simulink model "HANcoder_E407_DYS_MP"  (R2018b)
settings: Solver=FixedStepDiscrete  StartTime=0.0  StopTime=1  FixedStep=0.01  RelTol=1e-3
PreLoadFcn:
  | librarySetup
  | eval([bdroot,'_startup']) %Calling [modelName]_startup.m
values from neighbouring files (symbols this model uses):
  basic_cycle_duration_bc0 = TM_Reset_Board   + COMP_duration    (= 212)    [HANcoder_E407_DYS_MP_startup.m]
  basic_cycle_duration_bc1 = basic_cycle_duration_bc0    (= 212)    [HANcoder_E407_DYS_MP_startup.m]
  comm_delay_estimation1 = round(comm_delay_measured1*hardware_granularity/frequency_IRQ)    [HANcoder_E407_DYS_MP_startup.m]
  comm_delay_estimation2 = round(comm_delay_measured2*hardware_granularity/frequency_IRQ)    [HANcoder_E407_DYS_MP_startup.m]
  COMM_Phase1 = Simulink.Parameter    [HANcoder_E407_DYS_MP_startup.m]
  COMM_Phase2 = Simulink.Parameter    [HANcoder_E407_DYS_MP_startup.m]
  frequency_IRQ = 500    [HANcoder_E407_DYS_MP_startup.m]
  HantuneAngleSp = Simulink.Parameter    [HANcoder_E407_DYS_MP_startup.m]
  idle_time_init = basic_cycle_duration_bc0 + basic_cycle_duration_bc1    (= 424)    [HANcoder_E407_DYS_MP_startup.m]
  matrix_rows = 2    [HANcoder_E407_DYS_MP_startup.m]
  positionD = Simulink.Parameter    [HANcoder_E407_DYS_MP_startup.m]
  positionI = Simulink.Parameter    [HANcoder_E407_DYS_MP_startup.m]
  positionP = Simulink.Parameter    [HANcoder_E407_DYS_MP_startup.m]
undefined symbols (not defined in the file or in its folder): A1, CON2, CON4, D13, Dposition, Iposition, Pposition
libraries: HANcoder_STM32_Target x33, dspswit3 x16, simulink x2, simulink_extras x2, dspstat3 x1
(part 2 of 10)

== system HANcoder_E407_DYS_MP/HANcoder STM32 Target - E407-STM32 algorithm/4.TTA Can System/4.3 TTA System/4.3.1 Initialization/Receive can message ==
  Can_ID : Inport
  Action Port : ActionPort  ActionType=then
  CAN receive : Subsystem  Tag=HANcoder_TARGET_STM32_E407  AncestorBlock=HANcoder_STM32_Target/STM32-E407/CAN/CAN/CAN receive  mask(CAN receive){canBus=CAN 1, outputNumber=1, dataType=uint8, byteOrder=off, tsamp=-1}
      mask prompts: canBus "CAN channel"; outputNumber "Output ports"; dataType "Output datatype"; byteOrder "Byte order: Checked = MSB first, unchecked = LSB first."; tsamp "Sample time"
      mask help:
      | Function
      | ==========
      | Receive the newest message from the specified CAN channel.
      |
      | Parameters
      | ==========
      | CAN channel:             The CAN channel to send the message on.
      | Output ports:             The amount of output ports
      | Output datatype:       The datatype of the output ports
      | Byte order:                 Select MSB or LSB first
      | Sample time:              -1 or divisible by base sample time [seconds]
      |
      | Input
      | ==========
      | Port 1:                       CAN ID(uint32) in hexadecimal ie: hex2dec('0a')
      |
      | Output
      | ==========
      | Port 1:                       Checks for new message(int8)
      | Port 2..9                     Message data
      mask init:
      | sfcn_can_receive_mcb(canBus, outputNumber, dataType, byteOrder)
      settings: MoveFcn=drawLogos
      mask Help: web('sfcn_can_receive.html');
      mask TypeOptions canBus: CAN 1 | CAN 2
      mask TypeOptions dataType: int8 | uint8 | int16 | uint16 | int32 | uint32 | boolean
      mask Display:
      | fprintf('Receive on\nCAN %x', canBus);
      | port_label('output', 1, 'new');
      | port_label('input', 1, 'ID');patch([75 81 81],[8 14 2],[1 0 0]);patch([83 83 89],[14 2 8],[0 0 0.35]);
  CAN receive2 : Subsystem  Tag=HANcoder_TARGET_STM32_E407  AncestorBlock=HANcoder_STM32_Target/STM32-E407/CAN/CAN/CAN receive  mask(CAN receive){canBus=CAN 2, outputNumber=1, dataType=uint8, byteOrder=off, tsamp=-1}
      mask prompts: canBus "CAN channel"; outputNumber "Output ports"; dataType "Output datatype"; byteOrder "Byte order: Checked = MSB first, unchecked = LSB first."; tsamp "Sample time"
      mask help:
      | Function
      | ==========
      | Receive the newest message from the specified CAN channel.
      |
      | Parameters
      | ==========
      | CAN channel:             The CAN channel to send the message on.
      | Output ports:             The amount of output ports
      | Output datatype:       The datatype of the output ports
      | Byte order:                 Select MSB or LSB first
      | Sample time:              -1 or divisible by base sample time [seconds]
      |
      | Input
      | ==========
      | Port 1:                       CAN ID(uint32) in hexadecimal ie: hex2dec('0a')
      |
      | Output
      | ==========
      | Port 1:                       Checks for new message(int8)
      | Port 2..9                     Message data
      mask init:
      | sfcn_can_receive_mcb(canBus, outputNumber, dataType, byteOrder)
      settings: MoveFcn=drawLogos
      mask Help: web('sfcn_can_receive.html');
      mask TypeOptions canBus: CAN 1 | CAN 2
      mask TypeOptions dataType: int8 | uint8 | int16 | uint16 | int32 | uint32 | boolean
      mask Display:
      | fprintf('Receive on\nCAN %x', canBus);
      | port_label('output', 1, 'new');
      | port_label('input', 1, 'ID');patch([75 81 81],[8 14 2],[1 0 0]);patch([83 83 89],[14 2 8],[0 0 0.35]);
  Can1Mes1 : Outport
  Can1Receive : Outport  Port=2
  Can2Mes2 : Outport  Port=3
  Can2Receive : Outport  Port=4
  wires:
  CAN receive/2(Out2) -> Can1Mes1/1  "Test_CanMes0"
  CAN receive/1(Out1) -> Can1Receive/1  "Test_CanRec529"
  Can_ID/1 -> CAN receive2/1(In1), CAN receive/1(In1)
  CAN receive2/1(Out1) -> Can2Receive/1  "Test_Can2Rec529"
  CAN receive2/2(Out2) -> Can2Mes2/1  "Test_CanMes2"

== system HANcoder_E407_DYS_MP/HANcoder STM32 Target - E407-STM32 algorithm/4.TTA Can System/4.3 TTA System/4.3.1 Initialization/RoleID and Global Time init ==
  note: Reset variables
  note: Finish Initialization
  note: Role_ID Initialization
  Timeout Initialization : Inport
  Reference message received : Inport  Port=2
  Can1_Mes : Inport  Port=3
  Can1_New : Inport  Port=4
  Can2_Mes1 : Inport  Port=5
  Can2_New : Inport  Port=6
  Enable : EnablePort
  Constant : Constant  Priority=4
  Constant1 : Constant  Priority=3  Value=2
  Data Store Read : DataStoreRead  Priority=5  DataStoreName=Role_ID
  Data Store Write : DataStoreWrite  Priority=8  DataStoreName=Role_ID
  Data Store Write2 : DataStoreWrite  Priority=18  DataStoreName=Delay_Counter
  Data Store Write4 : DataStoreWrite  Priority=16  DataStoreName=Initialization_Timeout
  Global Time Initialization Master : Subsystem  Priority=2
  Global Time Initialization Slave : Subsystem  Priority=1
  RESET : Constant  Priority=15  Value=0  OutDataTypeStr=boolean
  RESET1 : Constant  Priority=17  Value=0  OutDataTypeStr=double
  SET : Constant  Priority=19
  Switch1 : Switch  Priority=6  Criteria=u2 > Threshold
  Switch2 : Switch  Priority=7  Criteria=u2 > Threshold
  Finish Initialization : Outport  OutputWhenDisabled=reset  InitialOutput=0
  wires:
  Switch1/1 -> Switch2/3
  Reference message received/1 -> Switch2/2, Global Time Initialization Slave/Enable  "Check"
  Data Store Read/1 -> Switch1/3
  SET/1 -> Finish Initialization/1
  Constant/1 -> Switch1/1
  Constant1/1 -> Switch2/1
  Switch2/1 -> Data Store Write/1
  RESET/1 -> Data Store Write4/1
  Timeout Initialization/1 -> Switch1/2, Global Time Initialization Master/Enable
  RESET1/1 -> Data Store Write2/1
  Can1_Mes/1 -> Global Time Initialization Slave/1(Can1_Mes)
  Can1_New/1 -> Global Time Initialization Slave/2(Can1_New)
  Can2_Mes1/1 -> Global Time Initialization Slave/3(Can2_Mes1)
  Can2_New/1 -> Global Time Initialization Slave/4(Can2_New)

== system HANcoder_E407_DYS_MP/HANcoder STM32 Target - E407-STM32 algorithm/4.TTA Can System/4.3 TTA System/4.3.3 Matrix Cycle Manager/4.3.3.1 Controller Matrix Cycle Truck Boards 1 2 and 3 ==
  note: Nodes Voting
      | Own_Vote:
      |    Individual vote of current node
      |
      |
      | Votes_count:
      |    Count of all received votes
  Enable : EnablePort  PropagateVarSize=During execution
  4.3.3.1.1 controller basic cycle 0.1 : Subsystem
  4.3.3.1.2 controller basic cycle 0.2 : Subsystem
  Data Store Memory : DataStoreMemory  DataStoreName=msg_count_DEBUG  ReadBeforeWriteMsg=warning  WriteAfterWriteMsg=warning  WriteAfterReadMsg=warning  ShowAdditionalParam=off
  Data Store Memory1 : DataStoreMemory  DataStoreName=Board1_error_counter  ReadBeforeWriteMsg=warning  WriteAfterWriteMsg=warning  WriteAfterReadMsg=warning  ShowAdditionalParam=off  OutMin=0  OutMax=4294967294  OutDataTypeStr=double
  Data Store Memory10 : DataStoreMemory  DataStoreName=Sensor_missed_counter  ReadBeforeWriteMsg=warning  WriteAfterWriteMsg=warning  WriteAfterReadMsg=warning  ShowAdditionalParam=off  OutMin=0  OutMax=4294967294  OutDataTypeStr=double
  Data Store Memory11 : DataStoreMemory  DataStoreName=Out1_missed_counter  ReadBeforeWriteMsg=warning  WriteAfterWriteMsg=warning  WriteAfterReadMsg=warning  ShowAdditionalParam=off  OutMin=0  OutMax=4294967294  OutDataTypeStr=double
  Data Store Memory12 : DataStoreMemory  Priority=30  DataStoreName=Own_Vote  ReadBeforeWriteMsg=warning  WriteAfterWriteMsg=warning  WriteAfterReadMsg=warning  ShowAdditionalParam=off  OutDataTypeStr=uint8
  Data Store Memory13 : DataStoreMemory  DataStoreName=Sync_bc1_missed_counter  ReadBeforeWriteMsg=warning  WriteAfterWriteMsg=warning  WriteAfterReadMsg=warning  ShowAdditionalParam=off  OutMin=0  OutMax=4294967294  OutDataTypeStr=double
  Data Store Memory14 : DataStoreMemory  DataStoreName=Out2_missed_counter  ReadBeforeWriteMsg=warning  WriteAfterWriteMsg=warning  WriteAfterReadMsg=warning  ShowAdditionalParam=off  OutMin=0  OutMax=4294967294  OutDataTypeStr=double
  Data Store Memory15 : DataStoreMemory  DataStoreName=NoMes1Cnt  ReadBeforeWriteMsg=warning  WriteAfterWriteMsg=warning  WriteAfterReadMsg=warning  ShowAdditionalParam=off  OutMin=0  OutMax=4294967294  OutDataTypeStr=double
  Data Store Memory16 : DataStoreMemory  DataStoreName=NoMes2Cnt  ReadBeforeWriteMsg=warning  WriteAfterWriteMsg=warning  WriteAfterReadMsg=warning  ShowAdditionalParam=off  OutMin=0  OutMax=4294967294  OutDataTypeStr=double
  Data Store Memory17 : DataStoreMemory  DataStoreName=NoMes3Cnt  ReadBeforeWriteMsg=warning  WriteAfterWriteMsg=warning  WriteAfterReadMsg=warning  ShowAdditionalParam=off  OutMin=0  OutMax=4294967294  OutDataTypeStr=double
  Data Store Memory18 : DataStoreMemory  DataStoreName=CycleCnt  ReadBeforeWriteMsg=warning  WriteAfterWriteMsg=warning  WriteAfterReadMsg=warning  ShowAdditionalParam=off  OutMin=0  OutMax=4294967294  OutDataTypeStr=double
  Data Store Memory19 : DataStoreMemory  DataStoreName=VoteTime  ReadBeforeWriteMsg=warning  WriteAfterWriteMsg=warning  WriteAfterReadMsg=warning  ShowAdditionalParam=off  OutMin=0  OutMax=250  OutDataTypeStr=uint8
  Data Store Memory2 : DataStoreMemory  DataStoreName=Board2_error_counter  ReadBeforeWriteMsg=warning  WriteAfterWriteMsg=warning  WriteAfterReadMsg=warning  ShowAdditionalParam=off  OutMin=0  OutMax=4294967294  OutDataTypeStr=double
  Data Store Memory20 : DataStoreMemory  DataStoreName=NoMes1  ReadBeforeWriteMsg=warning  WriteAfterWriteMsg=warning  WriteAfterReadMsg=warning  ShowAdditionalParam=off  OutMin=0  OutMax=4294967294  OutDataTypeStr=double
  Data Store Memory21 : DataStoreMemory  DataStoreName=NoMes2  ReadBeforeWriteMsg=warning  WriteAfterWriteMsg=warning  WriteAfterReadMsg=warning  ShowAdditionalParam=off  OutMin=0  OutMax=4294967294  OutDataTypeStr=double
  Data Store Memory22 : DataStoreMemory  DataStoreName=NoMes3  ReadBeforeWriteMsg=warning  WriteAfterWriteMsg=warning  WriteAfterReadMsg=warning  ShowAdditionalParam=off  OutMin=0  OutMax=4294967294  OutDataTypeStr=double
  Data Store Memory3 : DataStoreMemory  DataStoreName=Board3_error_counter  ReadBeforeWriteMsg=warning  WriteAfterWriteMsg=warning  WriteAfterReadMsg=warning  ShowAdditionalParam=off  OutMin=0  OutMax=4294967294  OutDataTypeStr=double
  Data Store Memory4 : DataStoreMemory  Priority=30  DataStoreName=BC0_Vote2_processed  ReadBeforeWriteMsg=warning  WriteAfterWriteMsg=warning  WriteAfterReadMsg=warning  ShowAdditionalParam=off  OutDataTypeStr=boolean
  Data Store Memory5 : DataStoreMemory  Priority=30  DataStoreName=BC0_Vote3_processed  ReadBeforeWriteMsg=warning  WriteAfterWriteMsg=warning  WriteAfterReadMsg=warning  ShowAdditionalParam=off  OutDataTypeStr=boolean
  Data Store Memory6 : DataStoreMemory  Priority=30  DataStoreName=BC0_Vote1_processed  ReadBeforeWriteMsg=warning  WriteAfterWriteMsg=warning  WriteAfterReadMsg=warning  ShowAdditionalParam=off  OutDataTypeStr=boolean
  Data Store Memory7 : DataStoreMemory  DataStoreName=Sync_bc0_missed_counter  ReadBeforeWriteMsg=warning  WriteAfterWriteMsg=warning  WriteAfterReadMsg=warning  ShowAdditionalParam=off  OutMin=0  OutMax=4294967294  OutDataTypeStr=double
  Data Store Memory8 : DataStoreMemory  DataStoreName=Set_missed_counter  ReadBeforeWriteMsg=warning  WriteAfterWriteMsg=warning  WriteAfterReadMsg=warning  ShowAdditionalParam=off  OutMin=0  OutMax=4294967294  OutDataTypeStr=double
  Data Store Memory9 : DataStoreMemory  Priority=30  DataStoreName=Votes_count  ReadBeforeWriteMsg=warning  WriteAfterWriteMsg=warning  WriteAfterReadMsg=warning  ShowAdditionalParam=off  OutDataTypeStr=Bus: vote_array
  Matrix_Cycle_Observation_DEBUG : Subsystem
  msg_count_DEBUG observer : Subsystem

== system HANcoder_E407_DYS_MP/HANcoder STM32 Target - E407-STM32 algorithm/4.TTA Can System/4.3 TTA System/4.3.3 Matrix Cycle Manager/4.3.3.2 Controller Matrix Cycle_Board 4 and 5 ==
  Enable : EnablePort  PropagateVarSize=During execution
  controller basic cycle 0 : Subsystem
  controller basic cycle 0.2 : Subsystem

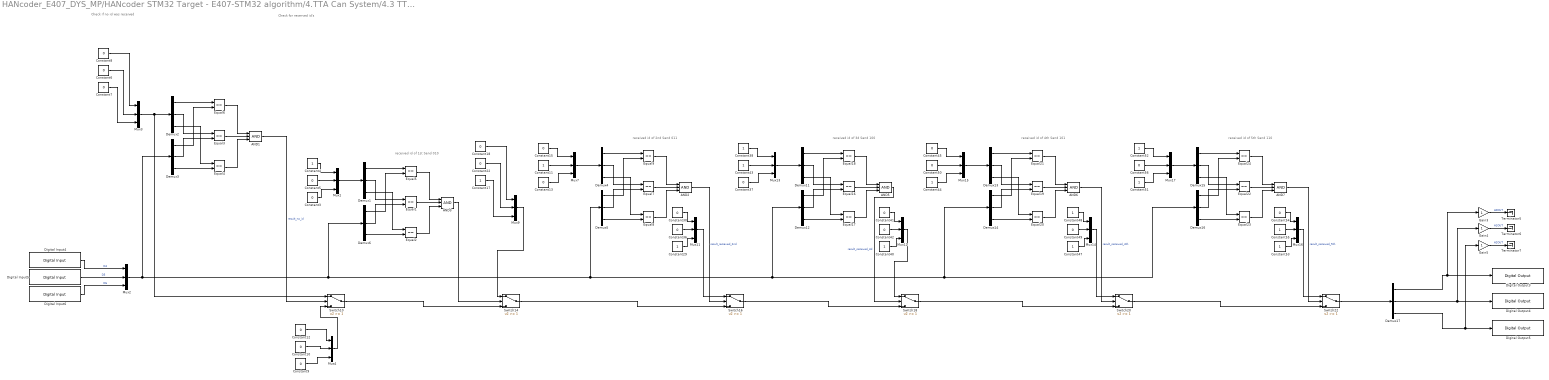
== system HANcoder_E407_DYS_MP/HANcoder STM32 Target - E407-STM32 algorithm/4.TTA Can System/4.3 TTA System/4.3.3 Matrix Cycle Manager/4.3.3.3 Send the next Board ID ==
  note: received id of 2nd
      | Send 011
  note: received id of 3d
      | Send 100
  note: received id of 4th
      | Send 101
  note: received id of 5th
      | Send 110
  note: Check if no id was received
  note: received id of 1st
      | Send 010
  note: Check for reserved id's
  AND{1..3,5..7} (6 alike) : Logic  Inputs=3  AllPortsSameDT=off  OutDataTypeStr=boolean
  Constant{3,5..10,12..13,15,18,22,30,36..37,41..42,45,49..50,54,56} (22 alike) : Constant  Value=0  OutDataTypeStr=boolean
  Constant{4,11,17,29,38,40,43..44,47..48,51..53,55} (14 alike) : Constant  OutDataTypeStr=boolean
  Demux{1..6,11..17} (13 alike) : Demux  Outputs=3
  Digital Input4 : HANcoder_STM32_Target/STM32-E407/Digital Inputs/Digital Input  Tag=HANcoder_TARGET_STM32_E407  pinID=CON3 - D2 - 5V Tolerant  config=Pulldown  tsamp=-1
      settings: SourceProductName=HANcoder STM32 Target
  Digital Input5 : HANcoder_STM32_Target/STM32-E407/Digital Inputs/Digital Input  Tag=HANcoder_TARGET_STM32_E407  pinID=CON3 - D3 - 5V Tolerant  config=Pulldown  tsamp=-1
      settings: SourceProductName=HANcoder STM32 Target
  Digital Input6 : HANcoder_STM32_Target/STM32-E407/Digital Inputs/Digital Input  Tag=HANcoder_TARGET_STM32_E407  pinID=CON3 - D4 - 5V Tolerant  config=Pulldown  tsamp=-1
      settings: SourceProductName=HANcoder STM32 Target
  Digital Output3 : HANcoder_STM32_Target/STM32-E407/Digital Outputs/Digital Output  Tag=HANcoder_TARGET_STM32_E407  pinID=CON PD - 8  config=Push pull  tsamp=-1
      settings: SourceProductName=HANcoder STM32 Target
  Digital Output4 : HANcoder_STM32_Target/STM32-E407/Digital Outputs/Digital Output  Tag=HANcoder_TARGET_STM32_E407  pinID=CON PD - 9  config=Push pull  tsamp=-1
      settings: SourceProductName=HANcoder STM32 Target
  Digital Output5 : HANcoder_STM32_Target/STM32-E407/Digital Outputs/Digital Output  Tag=HANcoder_TARGET_STM32_E407  pinID=CON PD - 10  config=Push pull  tsamp=-1
      settings: SourceProductName=HANcoder STM32 Target
  Equal{1..9,16..24} (18 alike) : RelationalOperator  Operator===  OutDataTypeStr=boolean  RndMeth=Simplest
  Gain3 : Gain
  Gain4 : Gain
  Gain5 : Gain
  Mux{1..4,7,9,11..17} (13 alike) : Mux  Inputs=3
  Switch{10,14,16,18,20,22} (6 alike) : Switch  Threshold=1
  Terminator5 : Terminator
  Terminator6 : Terminator
  Terminator7 : Terminator
  wires:
  Switch14/1 -> Switch16/3
  Constant29/1 -> Mux11/3
  Constant36/1 -> Mux11/2
  Constant17/1 -> Mux9/3
  Demux5/3 -> Equal8/2
  Mux9/1 -> Switch14/1
  Demux4/1 -> Equal9/1
  Demux5/2 -> Equal7/2
  Equal3/1 -> AND1/2
  Mux2/1 -> Demux3/1, Demux6/1, Demux5/1, Demux16/1, Demux14/1, Demux12/1
  Mux7/1 -> Demux4/1
  Demux4/2 -> Equal7/1
  Constant13/1 -> Mux7/3
  Demux2/2 -> Equal3/1
  Digital Input5/1 -> Mux2/2  "D5"
  Digital Input6/1 -> Mux2/3  "D6"
  Demux3/2 -> Equal3/2
  Constant41/1 -> Mux12/1
  AND2/1 -> Switch16/2  "result_recieved_2nd"
  Constant7/1 -> Mux3/3
  Constant51/1 -> Mux17/3
  Demux3/3 -> Equal4/2
  AND1/1 -> Switch10/2  "result_no_id"
  Demux15/2 -> Equal22/1
  Demux5/1 -> Equal9/2
  Switch22/1 -> Demux17/1
  Demux16/1 -> Equal24/2
  Equal9/1 -> AND2/1
  Mux15/1 -> Demux13/1
  Demux17/3 -> Gain5/1, Digital Output5/1
  Gain4/1 -> Terminator6/1  "A1OUT"
  Equal22/1 -> AND7/2
  Switch10/1 -> Switch14/3
  Constant12/1 -> Mux4/1
  Constant10/1 -> Mux4/2
  Constant9/1 -> Mux4/3
  Demux11/2 -> Equal16/1
  Demux14/1 -> Equal21/2
  Constant11/1 -> Mux7/2
  Switch18/1 -> Switch20/3
  Equal16/1 -> AND5/2
  Constant53/1 -> Mux16/3
  Equal6/1 -> AND1/1
  Demux12/1 -> Equal18/2
  Gain5/1 -> Terminator7/1  "A2OUT"
  Constant55/1 -> Mux16/2
  Mux16/1 -> Switch22/1
  Gain3/1 -> Terminator5/1  "A0OUT"
  Equal7/1 -> AND2/2
  Demux2/1 -> Equal6/1
  Demux15/3 -> Equal23/1
  Demux16/3 -> Equal23/2
  AND6/1 -> Switch20/2  "result_recieved_4th"
  Demux15/1 -> Equal24/1
  Switch20/1 -> Switch22/3
  Demux2/3 -> Equal4/1
  Demux16/2 -> Equal22/2
  Constant56/1 -> Mux17/2
  Mux14/1 -> Switch20/1
  Mux17/1 -> Demux15/1
  Demux17/1 -> Gain3/1, Digital Output3/1
  Constant37/1 -> Mux13/3
  Constant42/1 -> Mux12/2
  Constant6/1 -> Mux3/2
  Demux13/2 -> Equal19/1
  Demux4/3 -> Equal8/1
  Constant18/1 -> Mux9/1
  Constant8/1 -> Mux3/1
  Constant44/1 -> Mux15/3
  Constant49/1 -> Mux14/2
  Demux11/1 -> Equal18/1
  Constant47/1 -> Mux14/3
  Equal23/1 -> AND7/3
  Switch16/1 -> Switch18/3
  Constant40/1 -> Mux12/3
  Constant52/1 -> Mux17/1
  Constant38/1 -> Mux13/1
  Constant15/1 -> Mux7/1
  Constant22/1 -> Mux9/2
  Constant45/1 -> Mux15/1
  Equal4/1 -> AND1/3
  Mux3/1 -> Demux2/1, Switch10/1
  Mux11/1 -> Switch16/1
  Demux14/3 -> Equal20/2
  Demux12/3 -> Equal17/2
  Mux12/1 -> Switch18/1
  Equal24/1 -> AND7/1
  Demux11/3 -> Equal17/1
  Demux12/2 -> Equal16/2
  Equal19/1 -> AND6/2
  Demux13/3 -> Equal20/1
  AND5/1 -> Switch18/2  "result_recieved_3d"
  Demux17/2 -> Gain4/1, Digital Output4/1
  Constant43/1 -> Mux13/2
  Digital Input4/1 -> Mux2/1  "D4"
  Constant4/1 -> Mux1/1
  Equal17/1 -> AND5/3
  Demux14/2 -> Equal19/2
  Constant50/1 -> Mux15/2
  Demux3/1 -> Equal6/2
  Demux1/3 -> Equal2/1
  Constant54/1 -> Mux16/1
  Equal1/1 -> AND3/2
  Equal20/1 -> AND6/3
  Constant5/1 -> Mux1/2
  Equal2/1 -> AND3/3
  Constant3/1 -> Mux1/3
  Constant48/1 -> Mux14/1
  Demux1/2 -> Equal1/1
  Mux1/1 -> Demux1/1
  Constant30/1 -> Mux11/1
  Mux13/1 -> Demux11/1
  Equal18/1 -> AND5/1
  Demux1/1 -> Equal5/1
  AND7/1 -> Switch22/2  "result_recieved_5th"
  Demux6/3 -> Equal2/2
  Demux13/1 -> Equal21/1
  Equal21/1 -> AND6/1
  Demux6/1 -> Equal5/2
  Equal8/1 -> AND2/3
  Mux4/1 -> Switch10/3
  Demux6/2 -> Equal1/2
  Equal5/1 -> AND3/1
  AND3/1 -> Switch14/2

== system HANcoder_E407_DYS_MP/HANcoder STM32 Target - E407-STM32 algorithm/4.TTA Can System/4.3 TTA System/4.3.3 Matrix Cycle Manager/Matrix_Cycle_Observation_DEBUG ==
  Data Store Read1 : DataStoreRead  DataStoreName=TrailerOneAttachedFlag
  Data Store Read17 : DataStoreRead  DataStoreName=Votes_Angle  DataStoreElements=Votes_Angle.First_Board#Votes_Angle.Second_Board#Votes_Angle.Third_Board
  Data Store Read18 : DataStoreRead  DataStoreName=InputAngle1
  Data Store Read2 : DataStoreRead  DataStoreName=TwoTrailersAttachedFlag
  Data Store Read3 : DataStoreRead  DataStoreName=InputAngle2
  Data Store Read4 : DataStoreRead  DataStoreName=Votes_Encoder  DataStoreElements=Votes_Encoder.First_Board#Votes_Encoder.Second_Board#Votes_Encoder.Third_Board
  Terminator{1..6,19..22} (10 alike) : Terminator
  wires:
  Data Store Read18/1 -> Terminator22/1  "InputAngleBoard4"
  Data Store Read17/3 -> Terminator21/1  "VoteAngle3"
  Data Store Read17/2 -> Terminator20/1  "VoteAngle2"
  Data Store Read17/1 -> Terminator19/1  "VoteAngle1"
  Data Store Read1/1 -> Terminator1/1  "TrailerOneAttach"
  Data Store Read2/1 -> Terminator2/1  "TrailerTwoAttach"
  Data Store Read3/1 -> Terminator3/1  "InputAngleBoard5"
  Data Store Read4/1 -> Terminator4/1  "VoteEncoder1"
  Data Store Read4/3 -> Terminator6/1  "VoteEncoder3"
  Data Store Read4/2 -> Terminator5/1  "VoteEncoder2"

== system HANcoder_E407_DYS_MP/HANcoder STM32 Target - E407-STM32 algorithm/4.TTA Can System/4.3 TTA System/4.3.1 Initialization/Receive can message/CAN receive ==
  In1 : Inport
  Enabled Subsystem : Subsystem  TreatAsAtomicUnit=on
  S-Function : M-S-Function  FunctionName=sfcn_can_receive  Parameters=tsamp, canBus, outputNumber, dataType, byteOrder
  Term{3..9} (7 alike) : Terminator
  Out1 : Outport
  Out2 : Outport  Port=2
  wires:
  S-Function/9 -> Enabled Subsystem/8(In8)
  S-Function/4 -> Enabled Subsystem/3(In3)
  S-Function/5 -> Enabled Subsystem/4(In4)
  S-Function/8 -> Enabled Subsystem/7(In7)
  S-Function/7 -> Enabled Subsystem/6(In6)
  S-Function/6 -> Enabled Subsystem/5(In5)
  Enabled Subsystem/8(Out8) -> Term9/1
  Enabled Subsystem/7(Out7) -> Term8/1
  Enabled Subsystem/6(Out6) -> Term7/1
  Enabled Subsystem/5(Out5) -> Term6/1
  Enabled Subsystem/4(Out4) -> Term5/1
  Enabled Subsystem/3(Out3) -> Term4/1
  Enabled Subsystem/2(Out2) -> Term3/1
  Enabled Subsystem/1(Out1) -> Out2/1
  S-Function/3 -> Enabled Subsystem/2(In2)
  S-Function/2 -> Enabled Subsystem/1(In1)
  S-Function/1 -> Out1/1, Enabled Subsystem/Enable
  In1/1 -> S-Function/1

== system HANcoder_E407_DYS_MP/HANcoder STM32 Target - E407-STM32 algorithm/4.TTA Can System/4.3 TTA System/4.3.1 Initialization/Receive can message/CAN receive2 ==
  In1 : Inport
  Enabled Subsystem : Subsystem  TreatAsAtomicUnit=on
  S-Function : M-S-Function  FunctionName=sfcn_can_receive  Parameters=tsamp, canBus, outputNumber, dataType, byteOrder
  Term{3..9} (7 alike) : Terminator
  Out1 : Outport
  Out2 : Outport  Port=2
  wires:
  S-Function/9 -> Enabled Subsystem/8(In8)
  S-Function/4 -> Enabled Subsystem/3(In3)
  S-Function/5 -> Enabled Subsystem/4(In4)
  S-Function/8 -> Enabled Subsystem/7(In7)
  S-Function/7 -> Enabled Subsystem/6(In6)
  S-Function/6 -> Enabled Subsystem/5(In5)
  Enabled Subsystem/8(Out8) -> Term9/1
  Enabled Subsystem/7(Out7) -> Term8/1
  Enabled Subsystem/6(Out6) -> Term7/1
  Enabled Subsystem/5(Out5) -> Term6/1
  Enabled Subsystem/4(Out4) -> Term5/1
  Enabled Subsystem/3(Out3) -> Term4/1
  Enabled Subsystem/2(Out2) -> Term3/1
  Enabled Subsystem/1(Out1) -> Out2/1
  S-Function/3 -> Enabled Subsystem/2(In2)
  S-Function/2 -> Enabled Subsystem/1(In1)
  S-Function/1 -> Out1/1, Enabled Subsystem/Enable
  In1/1 -> S-Function/1

== system HANcoder_E407_DYS_MP/HANcoder STM32 Target - E407-STM32 algorithm/4.TTA Can System/4.3 TTA System/4.3.1 Initialization/RoleID and Global Time init/Global Time Initialization Master ==
  note: Global Time Initialization
  Enable : EnablePort
  Board nr1 : Constant
  Cast : DataTypeConversion  OutDataTypeStr=uint16
  Cast1 : DataTypeConversion  OutDataTypeStr=uint8
  Data Store Write : DataStoreWrite  DataStoreName=Local_Ticks
  Data Store Write1 : DataStoreWrite  DataStoreName=basic_cycle_count
  Data Store Write3 : DataStoreWrite  DataStoreName=Master_ID
  Start : Constant  Value=0
  wires:
  Board nr1/1 -> Data Store Write3/1
  Start/1 -> Cast1/1, Cast/1
  Cast/1 -> Data Store Write/1
  Cast1/1 -> Data Store Write1/1

== system HANcoder_E407_DYS_MP/HANcoder STM32 Target - E407-STM32 algorithm/4.TTA Can System/4.3 TTA System/4.3.1 Initialization/RoleID and Global Time init/Global Time Initialization Slave ==
  note: Sync has already been received, so we skip
      | the first comp tasks related to Update LT.
  note: Global Time Initialization
  Can1_Mes : Inport
  Can1_New : Inport  Port=2
  Can2_Mes1 : Inport  Port=3
  Can2_New : Inport  Port=4
  Enable : EnablePort
  Cast1 : DataTypeConversion  OutDataTypeStr=double
  Constant : Constant  Value=25  OutDataTypeStr=uint16
  Constant1 : Constant  Commented=on  Value=COMM_Phase1
  Constant2 : Constant  Commented=on  Value=COMM_Phase2
  Constant3 : Constant  Value=25  OutDataTypeStr=uint16
  Constant4 : Constant  Value=0  OutDataTypeStr=uint8
  Data Store Read : DataStoreRead  Priority=5  DataStoreName=Board_ID
  Data Store Write1 : DataStoreWrite  DataStoreName=Local_Ticks
  Data Store Write2 : DataStoreWrite  DataStoreName=basic_cycle_count
  Data Store Write3 : DataStoreWrite  DataStoreName=Master_ID
  Data Store Write4 : DataStoreWrite  Priority=10  DataStoreName=BC0_Sync_processed
  Data Type Conversion : DataTypeConversion  Commented=on  OutDataTypeStr=uint16
  Data Type Conversion1 : DataTypeConversion  Commented=on  OutDataTypeStr=uint16
  "SET1 " : Constant  Priority=9  OutDataTypeStr=boolean
  Sum : Sum  Priority=11  Inputs=+++  AccumDataTypeStr=uint16
  Sum1 : Sum  Priority=13  Inputs=+++  AccumDataTypeStr=uint16
  Switch1 : Switch  Priority=22  Criteria=u2 > Threshold
  delay_estimation_1 : Constant  Value=comm_delay_estimation1  OutDataTypeStr=uint16
  delay_estimation_2 : Constant  Value=comm_delay_estimation2  OutDataTypeStr=uint16
  wires:
  "SET1 "/1 -> Data Store Write4/1
  Switch1/1 -> Data Store Write1/1  "Rx_init_LT_Init"
  Cast1/1 -> Data Store Write3/1
  Constant/1 -> Sum/2
  delay_estimation_2/1 -> Sum1/3
  delay_estimation_1/1 -> Sum/3
  Can1_New/1 -> Switch1/2
  Sum/1 -> Switch1/1  "EstimatedTimeCan1_Init"
  Constant3/1 -> Sum1/2
  Sum1/1 -> Switch1/3  "EstimatedTimeCan2_Init"
  Constant4/1 -> Data Store Write2/1
  Data Store Read/1 -> Cast1/1
  Constant1/1 -> Data Type Conversion/1
  Data Type Conversion/1 -> Sum/1
  Constant2/1 -> Data Type Conversion1/1
  Data Type Conversion1/1 -> Sum1/1

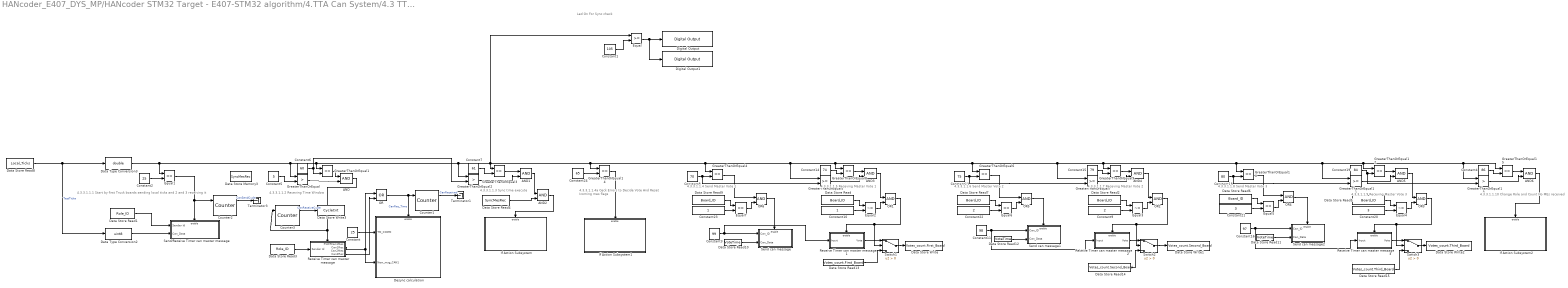
== system HANcoder_E407_DYS_MP/HANcoder STM32 Target - E407-STM32 algorithm/4.TTA Can System/4.3 TTA System/4.3.3 Matrix Cycle Manager/4.3.3.1 Controller Matrix Cycle Truck Boards 1 2 and 3/4.3.3.1.1 controller basic cycle 0.1 ==
  note: 4.3.3.1.1.1 Start by first Truck boards sending local ticks and 2 and 3 receiving it
  note: 4.3.3.1.1.2 Receving Time Window
  note: Led On For Sync check
  note: 4.3.3.1.1.3 Sync time execute
  note: 4.3.3.1.1.4 Send Master Vote 1
  note: 4.3.3.1.1.5 Receving Master Vote 1
  note: 4.3.3.1.1.6 Send Master Vote 2
  note: 4.3.3.1.1.7 Receving Master Vote 2
  note: 4.3.3.1.1.8 Send Master Vote 3
  note: 4.3.3.1.1.9 Receving Master Vote 3
  note: 4.3.3.1.1.4a Ceck Errors to Decide Vote
      | And Reset Icoming mes flags
  note: 4.3.3.1.1.10 Change Role and Count
      | No MEs received
  AND{,1..6} (7 alike) : Logic  IconShape=distinctive  AllPortsSameDT=off  OutDataTypeStr=boolean
  Constant : Constant  Value=25
  Constant1 : Constant  Value=105
  Constant10 : Constant
  Constant11 : Constant  Value=98  OutDataTypeStr=uint32
  Constant13 : Constant  Value=75
  Constant14 : Constant  Value=74
  Constant15 : Constant  Value=79
  Constant16 : Constant  Value=97  OutDataTypeStr=uint32
  Constant18 : Constant  Value=80
  Constant19 : Constant  Value=84
  Constant2 : Constant  Value=25
  Constant20 : Constant  Value=3
  Constant21 : Constant  Value=3
  Constant22 : Constant  Value=2
  Constant23 : Constant
  Constant24 : Constant  Value=65
  Constant3 : Constant  Value=99  OutDataTypeStr=uint32
  Constant4 : Constant  Value=86
  Constant5 : Constant  Value=5
  Constant6 : Constant  Value=60
  Constant7 : Constant  Value=61
  Constant8 : Constant  Value=70
  Constant9 : Constant  Value=2
  Counter1 : dspswit3/Counter  Direction=Up  CountEvent=Rising edge  CounterSize=User defined  MaxCount=255  InitialCount=0  Output=Count and Hit  HitValue=32  ResetInput=on  SamplesPerFrame=1  Ts=1  CntDtype=double  HitDtype=Logical
  Counter2 : dspswit3/Counter  Direction=Up  CountEvent=Rising edge  CounterSize=User defined  MaxCount=255  InitialCount=0  Output=Count and Hit  HitValue=32  ResetInput=on  SamplesPerFrame=1  Ts=1  CntDtype=double  HitDtype=Logical
  Counter3 : dspswit3/Counter  Direction=Up  CountEvent=Rising edge  CounterSize=User defined  MaxCount=255  InitialCount=0  Output=Count and Hit  HitValue=32  ResetInput=on  SamplesPerFrame=1  Ts=1  CntDtype=double  HitDtype=Logical
  Data Store Memory3 : DataStoreMemory  DataStoreName=SyncMesRec  ReadBeforeWriteMsg=warning  WriteAfterWriteMsg=warning  WriteAfterReadMsg=warning  ShowAdditionalParam=off  OutMin=0  OutMax=255  OutDataTypeStr=uint8
  Data Store Read{,2,5..7,9} (6 alike) : DataStoreRead  DataStoreName=Board_ID
  Data Store Read1 : DataStoreRead  Priority=10  DataStoreName=Role_ID
  Data Store Read10 : DataStoreRead  DataStoreName=VoteTime
  Data Store Read11 : DataStoreRead  DataStoreName=VoteTime
  Data Store Read12 : DataStoreRead  DataStoreName=VoteTime
  Data Store Read13 : DataStoreRead  DataStoreName=Votes_count  DataStoreElements=Votes_count.First_Board
  Data Store Read14 : DataStoreRead  DataStoreName=Votes_count  DataStoreElements=Votes_count.Second_Board
  Data Store Read15 : DataStoreRead  DataStoreName=Votes_count  DataStoreElements=Votes_count.Third_Board
  Data Store Read3 : DataStoreRead  Priority=10  DataStoreName=Role_ID
  Data Store Read4 : DataStoreRead  DataStoreName=SyncMesRec
  Data Store Read8 : DataStoreRead  DataStoreName=Local_Ticks
  Data Store Write : DataStoreWrite  DataStoreName=Votes_count  DataStoreElements=Votes_count.First_Board
  Data Store Write1 : DataStoreWrite  DataStoreName=Votes_count  DataStoreElements=Votes_count.Second_Board
  Data Store Write2 : DataStoreWrite  DataStoreName=Votes_count  DataStoreElements=Votes_count.Third_Board
  Data Store Write3 : DataStoreWrite  Priority=23  DataStoreName=CycleCnt
  Data Type Conversion2 : DataTypeConversion  OutDataTypeStr=uint8
  Data Type Conversion3 : DataTypeConversion  OutDataTypeStr=double
  Desync calculation : Subsystem  Priority=10
  Digital Output : HANcoder_STM32_Target/STM32-E407/Digital Outputs/Digital Output  Tag=HANcoder_TARGET_STM32_E407  pinID=CON4 - D13  config=Push pull  tsamp=-1
      settings: SourceProductName=HANcoder STM32 Target
  Digital Output1 : HANcoder_STM32_Target/STM32-E407/Digital Outputs/Digital Output  Tag=HANcoder_TARGET_STM32_E407  pinID=LED  config=Push pull  tsamp=-1
      settings: SourceProductName=HANcoder STM32 Target
  Equal : RelationalOperator  OutDataTypeStr=boolean  RndMeth=Simplest
  Equal{1,5..7} (4 alike) : RelationalOperator  Operator===  OutDataTypeStr=boolean  RndMeth=Simplest
  Equal2 : RelationalOperator  Operator=~=  OutDataTypeStr=boolean  RndMeth=Simplest
  Equal3 : RelationalOperator  Operator=~=  OutDataTypeStr=boolean  RndMeth=Simplest
  Equal4 : RelationalOperator  Operator=~=  OutDataTypeStr=boolean  RndMeth=Simplest
  GreaterThanOrEqual : RelationalOperator  Operator=>  OutDataTypeStr=boolean  RndMeth=Simplest
  GreaterThanOrEqual{1,3,8..9,12,15} (6 alike) : RelationalOperator  Operator=<=  OutDataTypeStr=boolean  RndMeth=Simplest
  GreaterThanOrEqual{4,6,10,14} (4 alike) : RelationalOperator  Operator===  OutDataTypeStr=boolean  RndMeth=Simplest
  GreaterThanOrEqual11 : RelationalOperator  OutDataTypeStr=boolean  RndMeth=Simplest
  GreaterThanOrEqual13 : RelationalOperator  Operator=>  OutDataTypeStr=boolean  RndMeth=Simplest
  GreaterThanOrEqual2 : RelationalOperator  Operator=>  OutDataTypeStr=boolean  RndMeth=Simplest
  GreaterThanOrEqual5 : RelationalOperator  OutDataTypeStr=boolean  RndMeth=Simplest
  GreaterThanOrEqual7 : RelationalOperator  OutDataTypeStr=boolean  RndMeth=Simplest
  If Action Subsystem : Subsystem  TreatAsAtomicUnit=on
  If Action Subsystem1 : Subsystem  TreatAsAtomicUnit=on
  If Action Subsystem2 : Subsystem  TreatAsAtomicUnit=on
  OR : Logic  Operator=OR  IconShape=distinctive  AllPortsSameDT=off  OutDataTypeStr=boolean
  OR{1..6} (6 alike) : Logic  IconShape=distinctive  AllPortsSameDT=off  OutDataTypeStr=boolean
  "Receive Timer can master message " : Subsystem
  Receive Timer can master message 1 : Subsystem
  Receive Timer can master message 2 : Subsystem
  Receive Timer can master message 3 : Subsystem
  Send can message : Subsystem  TreatAsAtomicUnit=on
  Send can message1 : Subsystem  TreatAsAtomicUnit=on
  Send can message2 : Subsystem  TreatAsAtomicUnit=on
  "Send/Receive Timer can master message " : Subsystem
  Switch1 : Switch  Criteria=u2 > Threshold
  Switch2 : Switch  Criteria=u2 > Threshold
  Switch3 : Switch  Criteria=u2 > Threshold
  Terminator1 : Terminator
  Terminator3 : Terminator
  wires:
  Data Store Read8/1 -> Data Type Conversion3/1, Data Type Conversion2/1  "TestTicka"
  Data Type Conversion2/1 -> "Send/Receive Timer can master message "/2(Can_Data)
  Data Store Read1/1 -> "Send/Receive Timer can master message "/1(Sender Id)
  Data Store Read3/1 -> "Receive Timer can master message "/1(Sender Id)
  Constant/1 -> Desync calculation/1(TM_COMM)
  "Receive Timer can master message "/2(Can1Rec) -> OR/1, Desync calculation/2(New_msg_CAN1)
  "Receive Timer can master message "/4(Can2Rec) -> OR/2
  OR/1 -> Counter1/1, Desync calculation/Enable  "CanRec_Time"
  Equal/1 -> Digital Output1/1, Digital Output/1
  Constant1/1 -> Equal/2
  Constant2/1 -> Equal1/2
  Equal1/1 -> Counter2/1, "Send/Receive Timer can master message "/Enable
  Constant5/1 -> GreaterThanOrEqual/2
  GreaterThanOrEqual/1 -> AND/2
  Constant6/1 -> GreaterThanOrEqual2/2, GreaterThanOrEqual1/2
  GreaterThanOrEqual1/1 -> AND/1
  Constant7/1 -> GreaterThanOrEqual3/2
  GreaterThanOrEqual3/1 -> AND1/1
  GreaterThanOrEqual2/1 -> AND1/2
  AND2/1 -> If Action Subsystem/Enable
  Counter1/1 -> Terminator1/1  "CanReceived"
  Counter2/1 -> Terminator3/1  "CanSendCycle"
  Counter3/1 -> Data Store Write3/1  "CanReceiveCycle"
  AND/1 -> Counter3/1, "Receive Timer can master message "/Enable
  AND1/1 -> AND2/1
  Data Store Read4/1 -> AND2/2
  Data Store Read10/1 -> Send can message/2(Can_Data)
  Constant8/1 -> GreaterThanOrEqual5/2, GreaterThanOrEqual4/2
  Equal2/1 -> OR1/2
  Data Store Read/1 -> Equal2/1
  Constant10/1 -> Equal2/2
  OR1/1 -> Switch1/2, Receive Timer can master message 1/Enable
  Constant3/1 -> Receive Timer can master message 1/1(Input), Send can message/1(Can_ID)
  OR2/1 -> Switch2/2, Receive Timer can master message 2/Enable
  Constant13/1 -> GreaterThanOrEqual7/2, GreaterThanOrEqual6/2
  Data Store Read2/1 -> Equal3/1
  Data Store Read12/1 -> Send can message1/2(Can_Data)
  Equal3/1 -> OR2/2
  Constant9/1 -> Equal3/2
  Constant11/1 -> Receive Timer can master message 2/1(Input), Send can message1/1(Can_ID)
  Constant14/1 -> GreaterThanOrEqual8/2
  GreaterThanOrEqual8/1 -> AND3/1
  GreaterThanOrEqual5/1 -> AND3/2
  AND3/1 -> OR1/1
  Receive Timer can master message 1/1(Vote) -> Switch1/1
  Constant15/1 -> GreaterThanOrEqual9/2
  GreaterThanOrEqual9/1 -> AND4/1
  GreaterThanOrEqual7/1 -> AND4/2
  AND4/1 -> OR2/1
  Receive Timer can master message 2/1(Vote) -> Switch2/1
  Constant18/1 -> GreaterThanOrEqual11/2, GreaterThanOrEqual10/2
  GreaterThanOrEqual11/1 -> AND5/2
  Data Type Conversion3/1 -> Equal1/1, GreaterThanOrEqual/1, GreaterThanOrEqual1/1, GreaterThanOrEqual2/1, GreaterThanOrEqual14/1, GreaterThanOrEqual8/1, GreaterThanOrEqual11/1, GreaterThanOrEqual13/1, GreaterThanOrEqual15/1, GreaterThanOrEqual12/1, GreaterThanOrEqual10/1, GreaterThanOrEqual9/1, GreaterThanOrEqual7/1, GreaterThanOrEqual6/1, GreaterThanOrEqual5/1, GreaterThanOrEqual4/1, GreaterThanOrEqual3/1, Equal/1
  OR3/1 -> Switch3/2, Receive Timer can master message 3/Enable
  Receive Timer can master message 3/1(Vote) -> Switch3/1
  Constant16/1 -> Receive Timer can master message 3/1(Input), Send can message2/1(Can_ID)
  Data Store Read11/1 -> Send can message2/2(Can_Data)
  Constant20/1 -> Equal4/2
  Equal4/1 -> OR3/2
  AND5/1 -> OR3/1
  GreaterThanOrEqual12/1 -> AND5/1
  Data Store Read5/1 -> Equal4/1
  Constant19/1 -> GreaterThanOrEqual13/2, GreaterThanOrEqual12/2
  Equal5/1 -> OR4/2
  Constant21/1 -> Equal5/2
  Data Store Read6/1 -> Equal5/1
  OR4/1 -> Send can message2/Enable
  GreaterThanOrEqual10/1 -> OR4/1
  Equal6/1 -> OR5/2
  Constant22/1 -> Equal6/2
  Data Store Read7/1 -> Equal6/1
  GreaterThanOrEqual6/1 -> OR5/1
  OR5/1 -> Send can message1/Enable
  GreaterThanOrEqual4/1 -> OR6/1
  Data Store Read9/1 -> Equal7/1
  Constant23/1 -> Equal7/2
  Equal7/1 -> OR6/2
  OR6/1 -> Send can message/Enable
  Constant24/1 -> GreaterThanOrEqual14/2
  GreaterThanOrEqual14/1 -> If Action Subsystem1/Enable
  Constant4/1 -> GreaterThanOrEqual15/2
  AND6/1 -> If Action Subsystem2/Enable
  GreaterThanOrEqual15/1 -> AND6/1
  GreaterThanOrEqual13/1 -> AND6/2
  Switch1/1 -> Data Store Write/1
  Data Store Read13/1 -> Switch1/3
  Switch2/1 -> Data Store Write1/1
  Data Store Read14/1 -> Switch2/3
  Switch3/1 -> Data Store Write2/1
  Data Store Read15/1 -> Switch3/3
